simulink model "restapi_station1_task"  (Simulink 3.00)
undefined symbols (not defined in the file): application, json
libraries: mathlib x5, stringlib x2, speclib x1

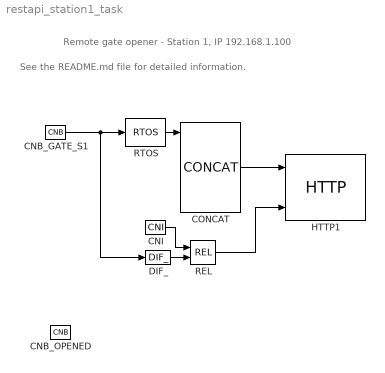
== system restapi_station1_task ==
  note: See the README.md file for detailed information.
  note: Remote gate opener - Station 1, IP 192.168.1.100
  CNB_GATE_S1 : mathlib/CNB  YCN=off
  CNB_OPENED : mathlib/CNB  YCN=off
  CNI : mathlib/CNI  icn=0
  CONCAT : stringlib/CONCAT  ptrn="{ \"v\": %1}"  nmax=0
  DIF_ : mathlib/DIF_
  HTTP1 : speclib/HTTP  url=http://192.168.1.200:8008/api/tasks/restapi_station2_task/CNB_GATE_S2:YCN  method=2  VERIFY=off  postmime=application/json  acceptmime=application/json  timeout=5  BLOCKING=off  nmax=0  postmax=256  datamax=1024
  REL : mathlib/REL  irel=2: inequality (!=)
  RTOS : stringlib/RTOS  prec=0  mode=1
  wires:
  CNB_GATE_S1/1 -> DIF_/1, RTOS/1
  CNI/1 -> REL/1
  CONCAT/1 -> HTTP1/1
  DIF_/1 -> REL/2
  REL/1 -> HTTP1/3
  RTOS/1 -> CONCAT/1
